simulink model "Sistema_Simulink"  (R2020a)
settings: Solver=ode45  StartTime=0.0  StopTime=30  FixedStep=0.0000000001  RelTol=1e-10  EnableMultiTasking=on
settings Model: Creator=kevinhmg  LastModifiedBy=gabri
settings DataIOCC: SaveFormat=Array  SignalLoggingSaveFormat=ModelDataLogs  ReturnWorkspaceOutputs=off  TimeSaveName=t
settings OptimizationCC: ExpressionDepthLimit=2147483647  LifeSpan=inf
settings DebuggingCC: UnderspecifiedInitializationDetection=Classic  MergeDetectMultiDrivingBlocksExec=none  SolverPrmCheckMsg=warning  FcnCallInpInsideContextMsg=warning  StateNameClashWarn=warning  SFUnexpectedBacktrackingDiag=warning  SFNoUnconditionalDefaultTransitionDiag=warning  SFExecutionAtInitializationDiag=none  ArithmeticOperatorsInVariantConditions=warning
settings HardwareCC: ProdBitPerPointer=32  ProdBitPerSizeT=32  ProdBitPerPtrDiffT=32  ProdLargestAtomicFloat=None  ProdIntDivRoundTo=Undefined  ProdEndianess=Unspecified  ProdWordSize=32  ProdHWDeviceType=32-bit Generic
settings ModelReferenceCC: PropagateSignalLabelsOutOfModel=off
settings SFSimCC: SimUseLocalCustomCode=off  CustomCodeUndefinedFunction=UseInterfaceOnly
settings RTWCC: RTWUseLocalCustomCode=off
settings CodeAppCC: StateflowObjectComments=on
settings GRTTargetCC: TargetLangStandard=C89/C90 (ANSI)  CombineOutputUpdateFcns=off  GRTInterface=on
settings ConfigComp: CovMetricSettings=dw  CovHtmlReporting=on  CovSaveCumulativeToWorkspaceVar=on  CovSaveSingleToWorkspaceVar=on  CovExternalEMLEnable=off

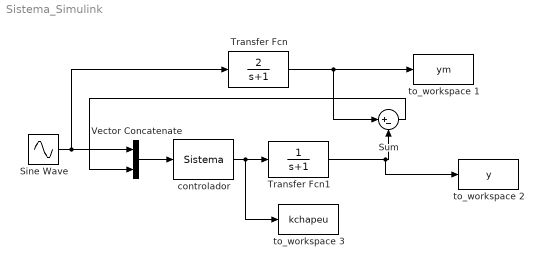
== system Sistema_Simulink ==
  Sine Wave : Sin  Amplitude=4  Frequency=1.884  SampleTime=0
  Sum : Sum  Inputs=|+-
  Transfer Fcn : TransferFcn  Numerator=[2]  Denominator=[1 1]
  Transfer Fcn1 : TransferFcn  Denominator=[1 1]
  Vector Concatenate : Concatenate
  controlador : S-Function  FunctionName=Sistema  SFunctionDeploymentMode=off  EnableBusSupport=off
  to_workspace 1 : ToWorkspace  VariableName=ym  SampleTime=-1
  to_workspace 2 : ToWorkspace  VariableName=y  SampleTime=-1
  to_workspace 3 : ToWorkspace  VariableName=kchapeu  SampleTime=-1
  wires:
  Transfer Fcn/1 -> to_workspace 1/1, Sum/1
  Vector Concatenate/1 -> controlador/1
  Transfer Fcn1/1 -> to_workspace 2/1, Sum/2
  controlador/1 -> to_workspace 3/1, Transfer Fcn1/1
  Sum/1 -> Vector Concatenate/2
  Sine Wave/1 -> Vector Concatenate/1, Transfer Fcn/1
